simulink model "LQG_controller2"  (R2016a)
settings: Solver=FixedStepDiscrete  SolverMode=SingleTasking  StartTime=0.0  StopTime=10  RelTol=1e-3
libraries: cstblocks x2
settings Model: Creator=Amir Rahmani  LastModifiedBy=kmoaz_000
settings OptimizationCC: DefaultParameterBehavior=Inlined  UseDivisionForNetSlopeComputation=on  UseFloatMulNetSlope=on  InlineInvariantSignals=on  PassReuseOutputArgsAs=Individual arguments  ZeroExternalMemoryAtStartup=off  ZeroInternalMemoryAtStartup=off  NoFixptDivByZeroProtection=on  EfficientFloat2IntCast=on  OptimizeModelRefInitCode=on  LifeSpan=1
settings RTWCC: SystemTargetFile=ert.tlc  GenCodeOnly=on  TemplateMakefile=ert_default_tmf  GenerateReport=on  IncludeHyperlinkInReport=on  LaunchReport=on  GenerateTraceInfo=on  GenerateTraceReport=on  GenerateTraceReportSl=on  GenerateTraceReportSf=on  GenerateTraceReportEml=on  GenerateCodeMetricsReport=on
settings CodeAppCC: ForceParamTrailComments=on  IgnoreCustomStorageClasses=off  OperatorAnnotations=on  SimulinkDataObjDesc=on  SFDataObjDesc=on  MATLABFcnDesc=on  CustomSymbolStrGlobalVar=rt$N$M  CustomSymbolStrType=$N$M  CustomSymbolStrFcn=$N$M$F  CustomSymbolStrMacro=$N$M  InsertBlockDesc=on  MATLABSourceComments=on
settings ERTTargetCC: GenerateSampleERTMain=on  IncludeMdlTerminateFcn=off  CombineSignalStateStructs=on  SuppressErrorStatus=on  SupportAbsoluteTime=off  SupportComplex=off  InlinedParameterPlacement=NonHierarchical  ERTCustomFileTemplate=example_file_process.tlc  ERTFilePackagingFormat=CompactWithDataFile

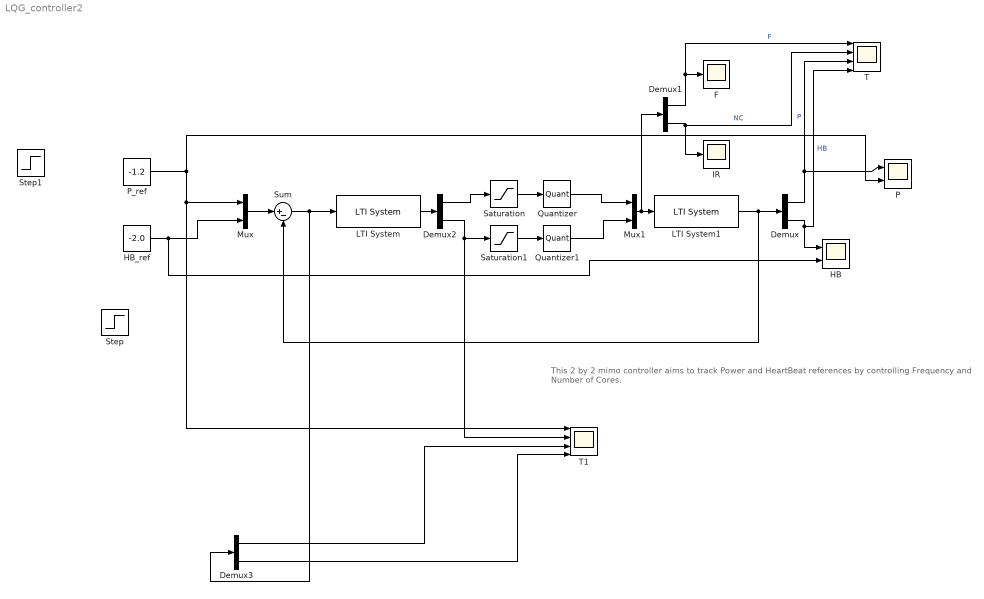
== system LQG_controller2 ==
  note: This 2 by 2 mimo controller aims to track Power and HeartBeat references by controlling Frequency and Number of Cores.
  Demux{,1..3} (4 alike) : Demux  Outputs=2
  F : Scope
  HB : Scope  NumInputPorts=2
  HB_ref : Constant  Value=-2.0
  IR : Scope
  LTI System : cstblocks/LTI System  sys=Klqg_mimo2x2  IC=[]
  LTI System1 : cstblocks/LTI System  sys=ss7  IC=[]
  Mux : Mux  Inputs=2
  Mux1 : Mux  Inputs=2
  P : Scope  NumInputPorts=2
  P_ref : Constant  Value=-1.2
  Quantizer : Quantizer  QuantizationInterval=0.1
  Quantizer1 : Quantizer  QuantizationInterval=1
  Saturation : Saturate  UpperLimit=0.4  LowerLimit=-0.4
  Saturation1 : Saturate  UpperLimit=2  LowerLimit=-2
  Step : Step  Before=.2  After=0  SampleTime=10
  Step1 : Step  Time=0  SampleTime=.05
  Sum : Sum  Inputs=|+-
  T : Scope  NumInputPorts=4
  T1 : Scope  NumInputPorts=4
  wires:
  P_ref/1 -> T1/1, Mux/1, P/2
  HB_ref/1 -> HB/2, Mux/2
  LTI System1/1 -> Sum/2, Demux/1
  Demux/1 -> T/3, P/1  "P"
  Demux/2 -> T/4, HB/1  "HB"
  Sum/1 -> Demux3/1, LTI System/1
  Demux1/1 -> T/1, F/1  "F"
  Demux1/2 -> T/2, IR/1  "NC"
  LTI System/1 -> Demux2/1
  Demux2/1 -> Saturation/1
  Mux1/1 -> Demux1/1, LTI System1/1
  Saturation/1 -> Quantizer/1
  Saturation1/1 -> Quantizer1/1
  Demux2/2 -> T1/2, Saturation1/1
  Demux3/1 -> T1/3
  Demux3/2 -> T1/4
  Mux/1 -> Sum/1
  Quantizer/1 -> Mux1/1
  Quantizer1/1 -> Mux1/2
